simulink model "SuperTwistingSlidingMode Voltage Control"  (R2023a)
settings: Solver=FixedStepAuto  StartTime=0.0  StopTime=5000  RelTol=1e-3
libraries: simulink_extras x8, matrix_library x4
settings Model: Creator=PC  LastModifiedBy=PC
settings SolverCC: ConcurrentTasks=on  PositivePriorityOrder=on
settings OptimizationCC: BlockReduction=off  OptimizeBlockIOStorage=off  BufferReuse=off  ZeroExternalMemoryAtStartup=off  ZeroInternalMemoryAtStartup=off
settings DebuggingCC: TasksWithSamePriorityMsg=none
settings HardwareCC: ProdBitPerLong=64  ProdLongLongMode=on  ProdHWDeviceType=Intel->x86-64 (Linux 64)
settings RTWCC: GenCodeOnly=on  Toolchain=Simulink Real-Time Toolchain  BuildConfiguration=Faster Runs  CodeExecutionProfiling=on  TargetLang=C++
settings GRTTargetCC: TargetLangStandard=C++03 (ISO)  CodeInterfacePackaging=C++ class

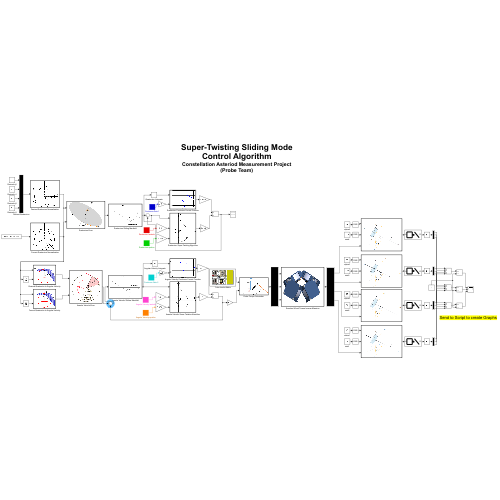
[thumbnail: Simulink's stored preview of the top-level diagram]
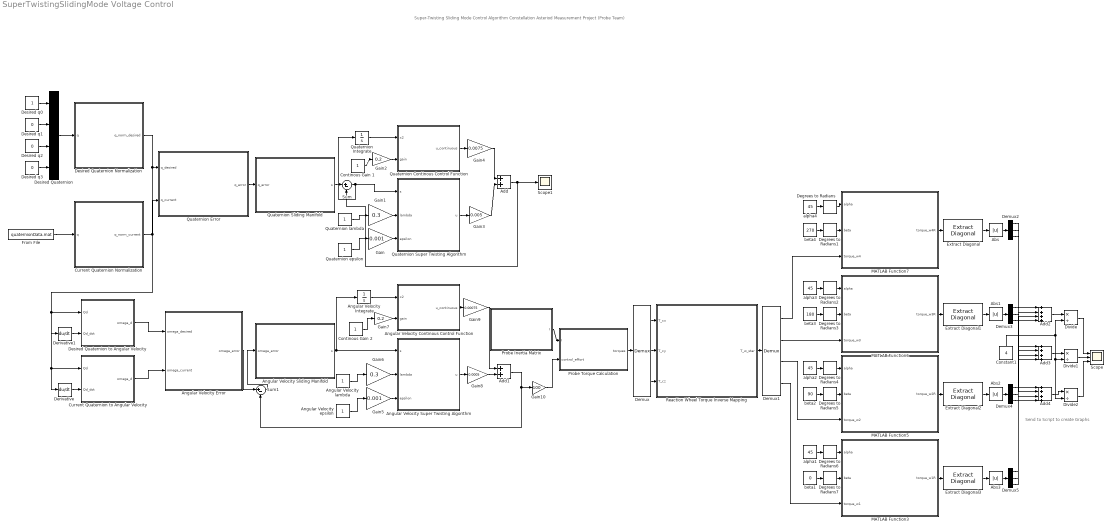
== system SuperTwistingSlidingMode Voltage Control ==
  note: Send to Script to create Graphs
  note: Super-Twisting Sliding Mode Control Algorithm
      | Constellation Asteriod Measurement Project
      | (Probe Team)
  Abs{,1..3} (4 alike) : Abs  SaturateOnIntegerOverflow=off
  Add : Sum
  Add1 : Sum
  Add2 : Sum  Inputs=++++
  Add3 : Sum  Inputs=++++
  Add4 : Sum  Inputs=++++
  Angular Velocity Continous Control Function : MATLAB Function  TreatAsAtomicUnit=on
  Angular Velocity Error : MATLAB Function  TreatAsAtomicUnit=on
  Angular Velocity Integrate : Integrator
  Angular Velocity Sliding Manifold : MATLAB Function  TreatAsAtomicUnit=on
  Angular Velocity Super Twisting Algorithm : MATLAB Function  TreatAsAtomicUnit=on
  Angular Velocity epsilon : Constant
  Angular Velocity lambda : Constant
  Constant1 : Constant  Value=4
  Continous Gain 1 : Constant
  Continous Gain 2 : Constant
  Current Quaternion Normalization : MATLAB Function  TreatAsAtomicUnit=on
  Current Quaternion to Angular Velocity : MATLAB Function  TreatAsAtomicUnit=on
  Degrees to Radians{,1..7} (8 alike) : simulink_extras/Transformations/Degrees to Radians
  Demux{,2..5} (5 alike) : Demux  Outputs=3
  Demux1 : Demux
  Derivative : Derivative
  Derivative1 : Derivative
  Desired Quaternion : Mux
  Desired Quaternion Normalization : MATLAB Function  TreatAsAtomicUnit=on
  Desired Quaternion to Angular Velocity : MATLAB Function  TreatAsAtomicUnit=on
  Desired q0 : Constant  SampleTime=0
  Desired q1 : Constant  Value=0  SampleTime=0
  Desired q2 : Constant  Value=0  SampleTime=0
  Desired q3 : Constant  Value=0  SampleTime=0
  Divide : Product  Inputs=*/
  Divide1 : Product  Inputs=*/
  Divide2 : Product  Inputs=*/
  Extract Diagonal{,1..3} (4 alike) : matrix_library/Extract Diagonal
      settings: LibrarySourceBlock=|
      | simulink/Matrix
      | Operations/Extract Diagonal
  From File : FromFile  FileName=quaternionData.mat  SampleTime=1
  Gain : Gain  Gain=0.001
  Gain1 : Gain  Gain=0.3
  Gain10 : Gain  Gain=100
  Gain2 : Gain  Gain=0.2
  Gain3 : Gain  Gain=0.005
  Gain4 : Gain  Gain=0.0075
  Gain5 : Gain  Gain=0.001
  Gain6 : Gain  Gain=0.3
  Gain7 : Gain  Gain=0.2
  Gain8 : Gain  Gain=0.0005
  Gain9 : Gain  Gain=0.00075
  MATLAB Function3 : MATLAB Function  TreatAsAtomicUnit=on
  MATLAB Function5 : MATLAB Function  TreatAsAtomicUnit=on
  MATLAB Function6 : MATLAB Function  TreatAsAtomicUnit=on
  MATLAB Function7 : MATLAB Function  TreatAsAtomicUnit=on
  Probe Inertia Matrix : Subsystem
      mask Display: image('C:\Users\PC\MATLAB\Picture1.png'); % Use "Edit Image" on toolstrip to change.
  Probe Torque Calculation : MATLAB Function  TreatAsAtomicUnit=on
  Quaternion Continous Control Function : MATLAB Function  TreatAsAtomicUnit=on
  Quaternion Error : MATLAB Function  TreatAsAtomicUnit=on
  Quaternion Integrate : Integrator
  Quaternion Sliding Manifold : MATLAB Function  TreatAsAtomicUnit=on
  Quaternion Super Twisting Algorithm : MATLAB Function  TreatAsAtomicUnit=on
  Quaternion epsilon : Constant
  Quaternion lambda : Constant
  Reaction Wheel Torque Inverse Mapping : MATLAB Function  TreatAsAtomicUnit=on
  Scope : Scope  NumInputPorts=3
  Scope1 : Scope
  Sum : Sum  Inputs=|+-
  Sum1 : Sum  Inputs=|+-
  alpha{1..4} (4 alike) : Constant  Value=45  SampleTime=0
  beta1 : Constant  Value=0
  beta2 : Constant  Value=90
  beta3 : Constant  Value=180
  beta4 : Constant  Value=270
  wires:
  Desired q3/1 -> Desired Quaternion/4
  Desired q2/1 -> Desired Quaternion/3
  Desired q1/1 -> Desired Quaternion/2
  Desired q0/1 -> Desired Quaternion/1
  Desired Quaternion/1 -> Desired Quaternion Normalization/1(q)
  From File/1 -> Current Quaternion Normalization/1(q)
  Quaternion Error/1(q_error) -> Quaternion Sliding Manifold/1(q_error)
  Quaternion Integrate/1 -> Quaternion Continous Control Function/1(x2)
  Quaternion epsilon/1 -> Gain/1
  Gain/1 -> Quaternion Super Twisting Algorithm/3(epsilon)
  Quaternion lambda/1 -> Gain1/1
  Gain1/1 -> Quaternion Super Twisting Algorithm/2(lambda)
  Quaternion Super Twisting Algorithm/1(u) -> Gain3/1
  Continous Gain 1/1 -> Gain2/1
  Gain2/1 -> Quaternion Continous Control Function/2(gain)
  Quaternion Continous Control Function/1(u_continuous) -> Gain4/1
  Gain3/1 -> Add/2
  Gain4/1 -> Add/1
  Current Quaternion to Angular Velocity/1(omega_d) -> Angular Velocity Error/2(omega_current)
  Desired Quaternion Normalization/1(q_norm_desired) -> Derivative1/1, Desired Quaternion to Angular Velocity/1(Qd), Quaternion Error/1(q_desired)
  Derivative1/1 -> Desired Quaternion to Angular Velocity/2(Qd_dot)
  Derivative/1 -> Current Quaternion to Angular Velocity/2(Qd_dot)
  Desired Quaternion to Angular Velocity/1(omega_d) -> Angular Velocity Error/1(omega_desired)
  Current Quaternion Normalization/1(q_norm_current) -> Quaternion Error/2(q_current), Derivative/1, Current Quaternion to Angular Velocity/1(Qd)
  Gain5/1 -> Angular Velocity Super Twisting Algorithm/3(epsilon)
  Angular Velocity Continous Control Function/1(u_continuous) -> Gain9/1
  Gain9/1 -> Add1/1
  Continous Gain 2/1 -> Gain7/1
  Angular Velocity epsilon/1 -> Gain5/1
  Gain6/1 -> Angular Velocity Super Twisting Algorithm/2(lambda)
  Angular Velocity Sliding Manifold/1(s) -> Angular Velocity Super Twisting Algorithm/1(s), Angular Velocity Integrate/1
  Angular Velocity lambda/1 -> Gain6/1
  Gain7/1 -> Angular Velocity Continous Control Function/2(gain)
  Gain8/1 -> Add1/2
  Angular Velocity Integrate/1 -> Angular Velocity Continous Control Function/1(x2)
  Angular Velocity Super Twisting Algorithm/1(u) -> Gain8/1
  Probe Torque Calculation/1(torques) -> Demux/1
  Demux/1 -> Reaction Wheel Torque Inverse Mapping/1(T_cx)
  Demux/2 -> Reaction Wheel Torque Inverse Mapping/2(T_cy)
  Demux/3 -> Reaction Wheel Torque Inverse Mapping/3(T_cz)
  Reaction Wheel Torque Inverse Mapping/1(T_w_star) -> Demux1/1
  Demux1/1 -> MATLAB Function7/3(torque_w4)
  Demux1/2 -> MATLAB Function6/3(torque_w3)
  Demux1/3 -> MATLAB Function5/3(torque_w2)
  Demux1/4 -> MATLAB Function3/3(torque_w1)
  Degrees to Radians/1 -> MATLAB Function7/1(alpha)
  alpha4/1 -> Degrees to Radians/1
  beta4/1 -> Degrees to Radians1/1
  Degrees to Radians1/1 -> MATLAB Function7/2(beta)
  alpha3/1 -> Degrees to Radians2/1
  Degrees to Radians2/1 -> MATLAB Function6/1(alpha)
  beta3/1 -> Degrees to Radians3/1
  Degrees to Radians3/1 -> MATLAB Function6/2(beta)
  alpha2/1 -> Degrees to Radians4/1
  Degrees to Radians4/1 -> MATLAB Function5/1(alpha)
  beta2/1 -> Degrees to Radians5/1
  Degrees to Radians5/1 -> MATLAB Function5/2(beta)
  alpha1/1 -> Degrees to Radians6/1
  Degrees to Radians6/1 -> MATLAB Function3/1(alpha)
  beta1/1 -> Degrees to Radians7/1
  Degrees to Radians7/1 -> MATLAB Function3/2(beta)
  Probe Inertia Matrix/1(I) -> Probe Torque Calculation/1(I)
  MATLAB Function7/1(torque_w4R) -> Extract Diagonal/1
  MATLAB Function3/1(torque_w1R) -> Extract Diagonal3/1
  MATLAB Function6/1(torque_w3R) -> Extract Diagonal1/1
  Extract Diagonal/1 -> Abs/1
  Abs/1 -> Demux2/1
  Abs1/1 -> Demux3/1
  Extract Diagonal1/1 -> Abs1/1
  Abs2/1 -> Demux4/1
  Extract Diagonal2/1 -> Abs2/1
  MATLAB Function5/1(torque_w2R) -> Extract Diagonal2/1
  Abs3/1 -> Demux5/1
  Extract Diagonal3/1 -> Abs3/1
  Demux2/1 -> Add2/1
  Demux3/1 -> Add2/2
  Demux4/1 -> Add2/3
  Demux5/1 -> Add2/4
  Add2/1 -> Divide/1
  Constant1/1 -> Divide/2, Divide2/2, Divide1/2
  Add3/1 -> Divide1/1
  Demux2/2 -> Add3/1
  Demux3/2 -> Add3/2
  Demux4/2 -> Add3/3
  Demux5/2 -> Add3/4
  Add4/1 -> Divide2/1
  Demux2/3 -> Add4/1
  Demux3/3 -> Add4/2
  Demux4/3 -> Add4/3
  Demux5/3 -> Add4/4
  Divide2/1 -> Scope/3
  Divide/1 -> Scope/1
  Divide1/1 -> Scope/2
  Quaternion Sliding Manifold/1(s) -> Sum/1
  Sum/1 -> Quaternion Integrate/1, Quaternion Super Twisting Algorithm/1(s)
  Add/1 -> Scope1/1, Sum/2
  Add1/1 -> Gain10/1, Sum1/2
  Angular Velocity Error/1(omega_error) -> Sum1/1
  Sum1/1 -> Angular Velocity Sliding Manifold/1(omega_error)
  Gain10/1 -> Probe Torque Calculation/2(control_effort)

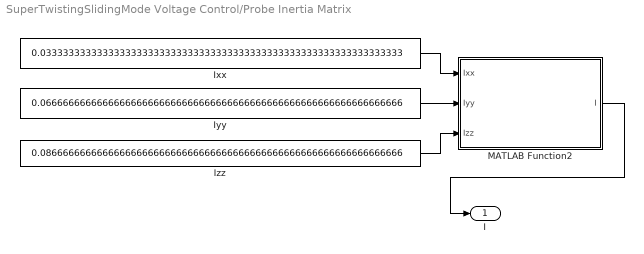
== system SuperTwistingSlidingMode Voltage Control/Probe Inertia Matrix ==
  Ixx : Constant  Value=0.0333333333333333333333333333333333333333333333333333333333333333  SampleTime=0
  Iyy : Constant  Value=0.0666666666666666666666666666666666666666666666666666666666666666  SampleTime=0
  Izz : Constant  Value=0.0866666666666666666666666666666666666666666666666666666666666666  SampleTime=0
  MATLAB Function2 : MATLAB Function  TreatAsAtomicUnit=on
  I : Outport
  wires:
  Izz/1 -> MATLAB Function2/3(Izz)
  Ixx/1 -> MATLAB Function2/1(Ixx)
  Iyy/1 -> MATLAB Function2/2(Iyy)
  MATLAB Function2/1(I) -> I/1

== matlab function SuperTwistingSlidingMode Voltage Control/Probe Torque Calculation ==
  data: I input; torques output; control_effort input
function torques = calcTorques(I, control_effort)
    % Compute torques
    torques = I * control_effort;
end

== matlab function SuperTwistingSlidingMode Voltage Control/Probe Inertia Matrix/MATLAB Function2 ==
  data: Ixx input; I output; Iyy input; Izz input
function I = inertiaMatrix(Ixx, Iyy, Izz)
    % Inertia Matrix for CubeSat
    I = [Ixx, 0, 0;
         0, Iyy, 0;
         0, 0, Izz];
end

== matlab function SuperTwistingSlidingMode Voltage Control/Reaction Wheel Torque Inverse Mapping ==
  data: T_cx input; T_w_star output; T_cy input; T_cz input
function T_w_star = mapTorquesToActuators(T_cx, T_cy, T_cz)
    % Define the transformation matrix
    M = (1/4) * [ sqrt(3),  sqrt(3),  sqrt(3),  1;
                  -sqrt(3),  sqrt(3),  sqrt(3), -1;
                  -sqrt(3), -sqrt(3),  sqrt(3),  1;
                   sqrt(3), -sqrt(3),  sqrt(3), -1];

    % Map the control torques to actuator torques
    T_w_star = M * [T_cx; T_cy; T_cz; 0];  % Note the zero for the fourth element since there is no τ_cz* term
end

== matlab function SuperTwistingSlidingMode Voltage Control/MATLAB Function3 ==
  data: alpha input; torque_w1R output; beta input; torque_w1 input
function torque_w1R = reactionWheelRotationMatrix_1(alpha, beta, torque_w1)
    % Compute the rotation matrix Ri for a single reaction wheel.
    % alpha: rotation angle around the y-axis
    % beta_i: tilt angle of the reaction wheel from the z-axis
    i = 1;
    pi = 3.1415926535897932384626433832795;
    beta_1 = beta + 0.5 * (i - 1) * pi;

    Ri_1 = [cos(alpha) * cos(beta_1),  cos(alpha) * sin(beta_1),  sin(alpha);
          -sin(beta_1),              cos(beta_1),              0;
          -cos(beta_1) * sin(alpha), -sin(alpha) * sin(beta_1), cos(alpha)];

    torque_w1R = torque_w1 * Ri_1;
end

== matlab function SuperTwistingSlidingMode Voltage Control/MATLAB Function5 ==
  data: alpha input; torque_w2R output; beta input; torque_w2 input
function torque_w2R = reactionWheelRotationMatrix_2(alpha, beta, torque_w2)
    % Compute the rotation matrix Ri for a single reaction wheel.
    % alpha: rotation angle around the y-axis
    % beta_i: tilt angle of the reaction wheel from the z-axis
    i = 2;
    pi = 3.1415926535897932384626433832795;
    beta_2 = beta + 0.5 * (i - 1) * pi;

    Ri_2 = [cos(alpha) * cos(beta_2),  cos(alpha) * sin(beta_2),  sin(alpha);
          -sin(beta_2),              cos(beta_2),              0;
          -cos(beta_2) * sin(alpha), -sin(alpha) * sin(beta_2), cos(alpha)];

    torque_w2R = torque_w2 * Ri_2;
end

== matlab function SuperTwistingSlidingMode Voltage Control/MATLAB Function6 ==
  data: alpha input; torque_w3R output; beta input; torque_w3 input
function torque_w3R = reactionWheelRotationMatrix_3(alpha, beta, torque_w3)
    % Compute the rotation matrix Ri for a single reaction wheel.
    % alpha: rotation angle around the y-axis
    % beta_i: tilt angle of the reaction wheel from the z-axis
    i = 3;
    pi = 3.1415926535897932384626433832795;
    beta_3 = beta + 0.5 * (i - 1) * pi;

    Ri_3 = [cos(alpha) * cos(beta_3),  cos(alpha) * sin(beta_3),  sin(alpha);
          -sin(beta_3),              cos(beta_3),              0;
          -cos(beta_3) * sin(alpha), -sin(alpha) * sin(beta_3), cos(alpha)];
    
    torque_w3R = torque_w3 * Ri_3;
end

== matlab function SuperTwistingSlidingMode Voltage Control/MATLAB Function7 ==
  data: alpha input; torque_w4R output; beta input; torque_w4 input
function torque_w4R = reactionWheelRotationMatrix_4(alpha, beta, torque_w4)
    % Compute the rotation matrix Ri for a single reaction wheel.
    % alpha: rotation angle around the y-axis
    % beta_i: tilt angle of the reaction wheel from the z-axis
    i = 4;
    pi = 3.1415926535897932384626433832795;
    beta_4 = beta + 0.5 * (i - 1) * pi;

    Ri_4 = [cos(alpha) * cos(beta_4),  cos(alpha) * sin(beta_4),  sin(alpha);
          -sin(beta_4),              cos(beta_4),              0;
          -cos(beta_4) * sin(alpha), -sin(alpha) * sin(beta_4), cos(alpha)];

    torque_w4R = torque_w4 * Ri_4;
end

== matlab function SuperTwistingSlidingMode Voltage Control/Desired Quaternion Normalization ==
  data: q input; q_norm_desired output
function q_norm_desired = normalizeQuaternion(q)
    % Calculate the norm (magnitude) of the quaternion
    norm_q = sqrt(q(1)^2 + q(2)^2 + q(3)^2 + q(4)^2);
    
    % Avoid division by zero by adding a small epsilon
    epsilon = 1e-10;
    if norm_q < epsilon
        norm_q = epsilon;
    end

    % Normalize the quaternion
    q_norm_desired = q / norm_q;
end

== matlab function SuperTwistingSlidingMode Voltage Control/Quaternion Error ==
  data: q_desired input; q_error output; q_current input
function q_error = quaternionError(q_desired, q_current)
    % Quaternion conjugate of the desired orientation
    q_conj = [q_desired(1), -q_desired(2), -q_desired(3), -q_desired(4)];
    
    % Quaternion multiplication: q_conj * q_current
    q_error = quatmultiply(q_conj, q_current);
end

function q_out = quatmultiply(q1, q2)
    % Multiplies two quaternions q1 and q2
    w1 = q1(1); x1 = q1(2); y1 = q1(3); z1 = q1(4);
    w2 = q2(1); x2 = q2(2); y2 = q2(3); z2 = q2(4);
    
    w = w1*w2 - x1*x2 - y1*y2 - z1*z2;
    x = w1*x2 + x1*w2 + y1*z2 - z1*y2;
    y = w1*y2 - x1*z2 + y1*w2 + z1*x2;
    z = w1*z2 + x1*y2 - y1*x2 + z1*w2;
    
    q_out = [w, x, y, z];
end

== matlab function SuperTwistingSlidingMode Voltage Control/Quaternion Sliding Manifold ==
  data: q_error input; s output
function s = calculateSlidingSurface(q_error)
    % Assuming the quaternion error is in the form [q0, q1, q2, q3]
    % and the scalar part q0 is the first element.

    % Extract the vector part of the quaternion error
    q_vector = q_error(2:4);
    
    % Calculate the sliding variable 's'
    % Here we just use the vector part directly, but in practice, this could
    % involve more complex operations based on the control requirements.
    s = q_vector;
end

== matlab function SuperTwistingSlidingMode Voltage Control/Quaternion Super Twisting Algorithm ==
  data: s input; u output; lambda input; epsilon input
function u = twistingControl(s, lambda, epsilon)
    % s: the sliding variable (vector part of quaternion error)
    % lambda: gain of the twisting control
    % epsilon: a small positive value to smooth the sign function
    
    % Check if epsilon is provided, otherwise set a default small value
    if nargin < 3
        epsilon = 0.01;  % Default small value to prevent division by zero
    end
    
    % Calculate the sign of s, treating zero as positive to avoid discontinuity at zero
    sgn_s = sign(s);
    sgn_s(sgn_s == 0) = 1;

    % Compute the control input u using the STA
    u = -sgn_s .* (lambda * sqrt(abs(s)) + epsilon);
end

== matlab function SuperTwistingSlidingMode Voltage Control/Quaternion Continous Control Function ==
  data: x2 input; u_continuous output; gain input
function u_continuous = continuousControl(x2, gain)
    % Simple proportional control using the integrated variable
    u_continuous = gain * x2;
end

== matlab function SuperTwistingSlidingMode Voltage Control/Current Quaternion to Angular Velocity ==
  data: Qd input; omega_d output; Qd_dot input
function omega_d = quatToAngularVel_current(Qd, Qd_dot)
    % Extract the quaternion elements
    q0d = Qd(1);
    q1d = Qd(2);
    q2d = Qd(3);
    q3d = Qd(4);

    % Define the E matrix for the desired quaternion
    E_Qd = [-q1d, -q2d, -q3d;
             q0d, -q3d,  q2d;
             q3d,  q0d, -q1d;
            -q2d,  q1d,  q0d];

    % Calculate the desired angular velocity
    omega_d = 2 * E_Qd' * Qd_dot;
end

== matlab function SuperTwistingSlidingMode Voltage Control/Angular Velocity Continous Control Function ==
  data: x2 input; u_continuous output; gain input
function u_continuous = continuousControl(x2, gain)
    % Simple proportional control using the integrated variable
    u_continuous = gain * x2;
end

== matlab function SuperTwistingSlidingMode Voltage Control/Angular Velocity Super Twisting Algorithm ==
  data: s input; u output; lambda input; epsilon input
function u = twistingControl(s, lambda, epsilon)
    % s: the sliding variable (vector part of quaternion error)
    % lambda: gain of the twisting control
    % epsilon: a small positive value to smooth the sign function
    
    % Check if epsilon is provided, otherwise set a default small value
    if nargin < 3
        epsilon = 0.01;  % Default small value to prevent division by zero
    end
    
    % Calculate the sign of s, treating zero as positive to avoid discontinuity at zero
    sgn_s = sign(s);
    sgn_s(sgn_s == 0) = 1;

    % Compute the control input u using the STA
    u = -sgn_s .* (lambda * sqrt(abs(s)) + epsilon);
end

== matlab function SuperTwistingSlidingMode Voltage Control/Desired Quaternion to Angular Velocity ==
  data: Qd input; omega_d output; Qd_dot input
function omega_d = quatToAngularVel_desired(Qd, Qd_dot)
    % Extract the quaternion elements
    q0d = Qd(1);
    q1d = Qd(2);
    q2d = Qd(3);
    q3d = Qd(4);

    % Define the E matrix for the desired quaternion
    E_Qd = [-q1d, -q2d, -q3d;
             q0d, -q3d,  q2d;
             q3d,  q0d, -q1d;
            -q2d,  q1d,  q0d];

    % Calculate the desired angular velocity
    omega_d = 2 * E_Qd' * Qd_dot;
end

== matlab function SuperTwistingSlidingMode Voltage Control/Angular Velocity Sliding Manifold ==
  data: omega_error input; s output
function s = calcSlidingManifold(omega_error)  
    % Calculate the sliding manifold
    s = omega_error;
end

== matlab function SuperTwistingSlidingMode Voltage Control/Current Quaternion Normalization ==
  data: q input; q_norm_current output
function q_norm_current = normalizeQuaternion(q)
    % Calculate the norm (magnitude) of the quaternion
    norm_q = sqrt(q(1)^2 + q(2)^2 + q(3)^2 + q(4)^2);
    
    % Avoid division by zero by adding a small epsilon
    epsilon = 1e-10;
    if norm_q < epsilon
        norm_q = epsilon;
    end

    % Normalize the quaternion
    q_norm_current = q / norm_q;
end

== matlab function SuperTwistingSlidingMode Voltage Control/Angular Velocity Error ==
  data: omega_desired input; omega_error output; omega_current input
function omega_error = omegaError(omega_desired, omega_current)
    % Calculate angular velocity error
    omega_error = omega_desired - omega_current;
end
